simulink model "LAB4_interface_demo"  (R2023b)
settings: Solver=FixedStepAuto  StartTime=0.0  StopTime=inf  FixedStep=0.01  RelTol=1e-3
undefined symbols (not defined in the file or in its folder): LF
libraries: instrumentseriallib x4, simulink x3, hdlsllib x1
settings Model: Creator=tanawatp  LastModifiedBy=Kitti

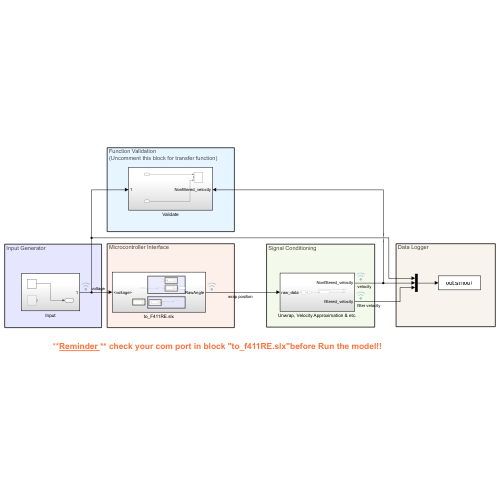
[thumbnail: Simulink's stored preview of the top-level diagram]
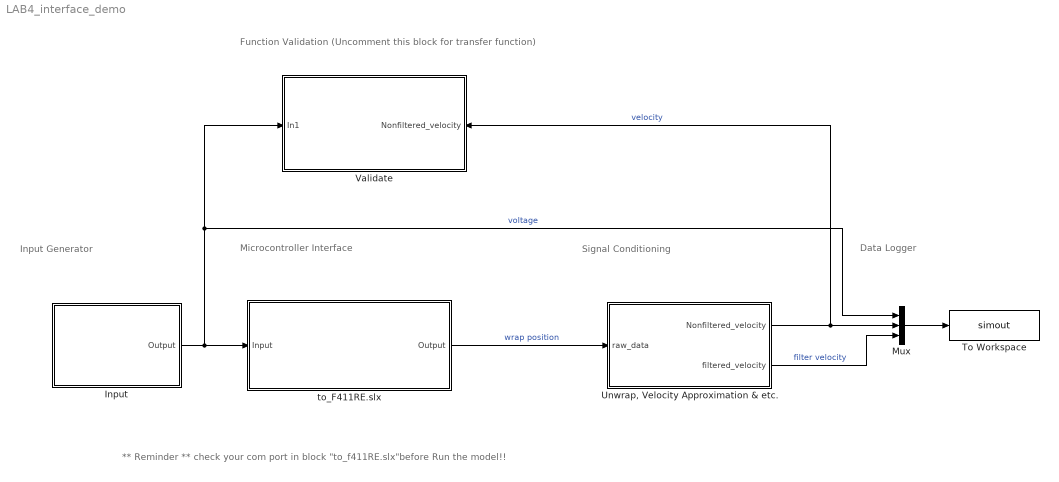
== system LAB4_interface_demo ==
  note: ** Reminder ** check your com port in block "to_f411RE.slx"before Run the model!!
  note: Signal Conditioning
  note: Function Validation
      | (Uncomment this block for transfer function)
  note: Input Generator
  note: Data Logger
  note: Microcontroller Interface
  Input : Subsystem
  Mux : Mux  Inputs=3
  To Workspace : ToWorkspace  VariableName=simout  SaveFormat=Timeseries  SampleTime=-1
  "Unwrap, Velocity Approximation & etc." : Subsystem
  Validate : Subsystem
      settings: PortSchema="{\"entries\":[{\"content\":{\"sides\":[{\"content\":{\"connectorIds\":[\"In1\"]},\"type\":\"ConnectorPlacement.EquallySpacedRectSide\",\"uuid\":\"2e198c62-3f63-40d2-bae8-9fd8fef67e0c\"},{\"content\":{\"connectorIds\":[\"In2\"],\"side\":\"RIGHT\"},\"type\":\"ConnectorPlacement.EquallySpacedRectSide\",\"uuid\":\"8587534e-14f7-4890-8a03-94178e65376b\"},{\"content\":{\"connectorIds\":[],\"side\":\"TOP\"},\"type\":\"ConnectorPlacement.EquallySpacedRectSide\",\"uuid\":\"1b7cad7c-cb5d-42c2-b7c5-a9278b867159\"}]},\"type\":\"ConnectorPlacement.EquallySpacedConnector\",\"uuid\":\"07c3edf9-7db3-4a0b-af16-87d57ef9c94a\"}],\"packageUris\":[\"http://schema.mathworks.com/mf0/Connector/R2020b\"],\"version\":\"1.0\"}"
  to_F411RE.slx : Subsystem
  wires:
  Mux/1 -> To Workspace/1
  to_F411RE.slx/1(Output) -> "Unwrap, Velocity Approximation & etc."/1(raw_data)  "wrap position"
  Input/1(Output) -> to_F411RE.slx/1(Input), Validate/1(In1), Mux/1  "voltage"
  "Unwrap, Velocity Approximation & etc."/1(Nonfiltered_velocity) -> Mux/2, Validate/2(Nonfiltered_velocity)  "velocity"
  "Unwrap, Velocity Approximation & etc."/2(filtered_velocity) -> Mux/3  "filter velocity"

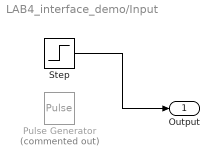
== system LAB4_interface_demo/Input ==
  Pulse Generator : DiscretePulseGenerator  Commented=on  PulseType=Time based  Amplitude=8  Period=5  PulseWidth=50  PhaseDelay=3
  Step : Step  After=6  SampleTime=0
  Output : Outport
  wires:
  Step/1 -> Output/1

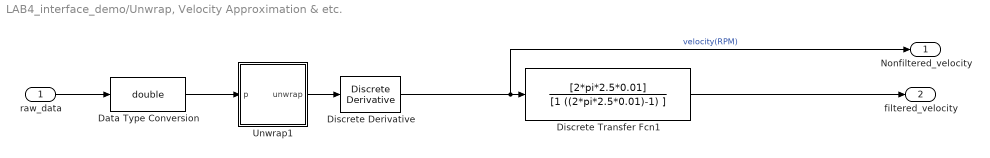
== system LAB4_interface_demo/Unwrap, Velocity Approximation & etc. ==
  raw_data : Inport
  Data Type Conversion : DataTypeConversion  OutDataTypeStr=double  SaturateOnIntegerOverflow=off  RndMeth=Floor
  Discrete Transfer Fcn1 : DiscreteTransferFcn  Numerator=[2*pi*2.5*0.01]  Denominator=[1 ((2*pi*2.5*0.01)-1) ]
  Discrete Derivative : simulink/Discrete/Discrete Derivative  gainval=60 / 4095  ICPrevScaledInput=0.0  OutMin=[]  OutMax=[]  OutDataType=fixdt(1, 16)  OutScaling=2^-10  DoSatur=off
  Unwrap1 : Subsystem
  Nonfiltered_velocity : Outport
  filtered_velocity : Outport  Port=2
  wires:
  Unwrap1/1(unwrap) -> Discrete Derivative/1
  raw_data/1 -> Data Type Conversion/1
  Discrete Transfer Fcn1/1 -> filtered_velocity/1
  Discrete Derivative/1 -> Nonfiltered_velocity/1, Discrete Transfer Fcn1/1  "velocity(RPM)"
  Data Type Conversion/1 -> Unwrap1/1(p)

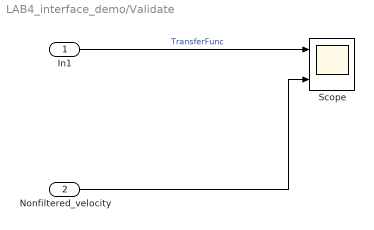
== system LAB4_interface_demo/Validate ==
  In1 : Inport
  Nonfiltered_velocity : Inport  Port=2
  Scope : Scope  NumInputPorts=3
  wires:
  Nonfiltered_velocity/1 -> Scope/3
  In1/1 -> Scope/1  "TransferFunc"

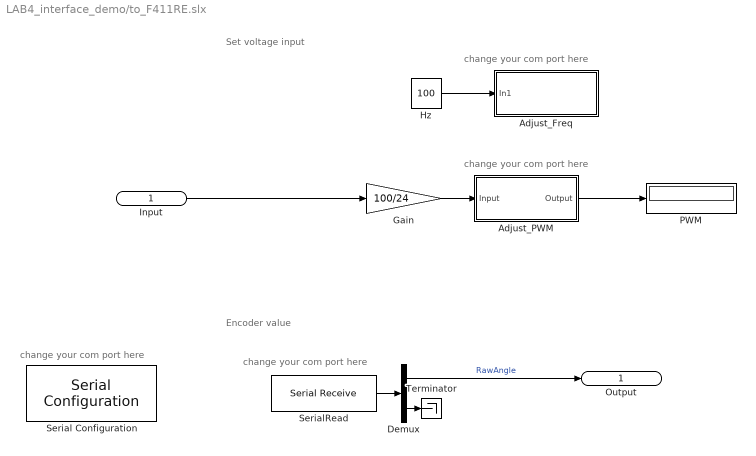
== system LAB4_interface_demo/to_F411RE.slx ==
  note: change your com port here
  note: Encoder value
  note: Set voltage input
  note: change your com port here
  note: change your com port here
  note: change your com port here
  Input : Inport
  Adjust_Freq : Subsystem
  Adjust_PWM : Subsystem
  Demux : Demux  Outputs=2
  Gain : Gain  Gain=100/24  OutDataTypeStr=int8
  Hz : Constant  Value=100  OutDataTypeStr=double
  PWM : Display
  Serial Configuration : instrumentseriallib/Serial Configuration  Priority=-200000  PortSel=COM5  Port=COM5  ComPort=COM5  BaudRate=115200  DataBits=8  Parity=none  StopBits=1  ByteOrder=little-endian  FlowControl=none  Timeout=10  SimulateUsing=Interpreted execution  BlockInModel=on  aMode=1
  SerialRead : instrumentseriallib/Serial Receive  Priority=1  PortSel=COM5  Port=COM5  ComPort=COM5  DataType=uint16  SaveDataType=uint8  ToggleHeader=on  Header=[69]  ToggleTerminator=on  Terminator=LF ('\n')  CustomTerminator=[]  InputFormat=Column major  ToggleDataSize=on  DataSize=[2]  EnableBlockingMode=on  ActionDataUnavailable=Output last received value  ActionWhenDataUnavailable=Output last received value  CustomValue=0  SampleTime=-1  SimulateUsing=Interpreted execution  BlockInModel=on  aMode=1
  Terminator : Terminator
  Output : Outport
  wires:
  Demux/1 -> Output/1  "RawAngle"
  Gain/1 -> Adjust_PWM/1(Input)
  Input/1 -> Gain/1
  Hz/1 -> Adjust_Freq/1(In1)
  Adjust_PWM/1(Output) -> PWM/1
  SerialRead/1 -> Demux/1
  Demux/2 -> Terminator/1

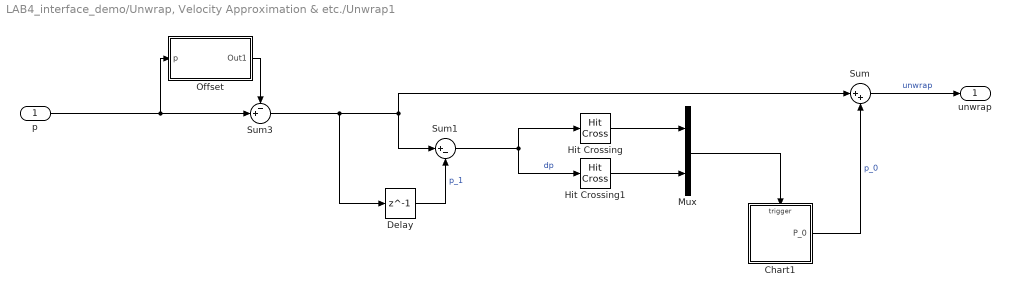
== system LAB4_interface_demo/Unwrap, Velocity Approximation & etc./Unwrap1 ==
  p : Inport
  Chart1 : Stateflow chart  TreatAsAtomicUnit=on
  Delay : Delay  DelayLength=1
  Hit Crossing : HitCross  HitCrossingOffset=0.7*65535  HitCrossingDirection=rising
  Hit Crossing1 : HitCross  HitCrossingOffset=-0.7*65535  HitCrossingDirection=falling
  Mux : Mux  Inputs=2
  Offset : Subsystem
  Sum : Sum  Inputs=|++
  Sum1 : Sum  Inputs=|+-
  Sum3 : Sum  Inputs=-+|
  unwrap : Outport
  wires:
  Hit Crossing/1 -> Mux/1
  Hit Crossing1/1 -> Mux/2
  Chart1/1(P_0) -> Sum/2  "p_0"
  Sum1/1 -> Hit Crossing1/1, Hit Crossing/1  "dp"
  Sum3/1 -> Delay/1, Sum/1, Sum1/1
  Mux/1 -> Chart1/Trigger
  Sum/1 -> unwrap/1  "unwrap"
  Delay/1 -> Sum1/2  "p_1"
  Offset/1(Out1) -> Sum3/1
  p/1 -> Sum3/2, Offset/1(p)

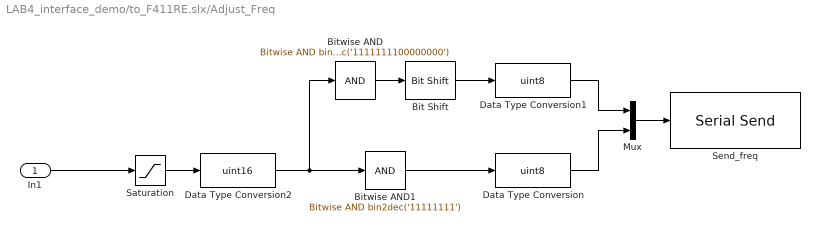
== system LAB4_interface_demo/to_F411RE.slx/Adjust_Freq ==
  In1 : Inport
  Bit Shift : hdlsllib/Logic and Bit Operations/Bit Shift  mode=Shift Right Logical  N=8
  Bitwise AND : simulink/Logic and Bit Operations/Bitwise Operator  logicop=AND  UseBitMask=on  BitMask=bin2dec('1111111100000000')  BitMaskRealWorld=Stored Integer
  Bitwise AND1 : simulink/Logic and Bit Operations/Bitwise Operator  logicop=AND  UseBitMask=on  BitMask=bin2dec('11111111')  BitMaskRealWorld=Stored Integer
  Data Type Conversion : DataTypeConversion  OutDataTypeStr=uint8  SaturateOnIntegerOverflow=off  RndMeth=Floor
  Data Type Conversion1 : DataTypeConversion  OutDataTypeStr=uint8  SaturateOnIntegerOverflow=off  RndMeth=Floor
  Data Type Conversion2 : DataTypeConversion  OutDataTypeStr=uint16  SaturateOnIntegerOverflow=off  RndMeth=Floor
  Mux : Mux  Inputs=2
  Saturation : Saturate  UpperLimit=20000  LowerLimit=5
  Send_freq : instrumentseriallib/Serial Send  Priority=1  PortSel=COM5  Port=COM5  ComPort=COM5  Header=[69]  Terminator=<none>  CustomTerminator=[123]  EnableBlockingMode=on  SimulateUsing=Interpreted execution  BlockInModel=on  aMode=1
  wires:
  Mux/1 -> Send_freq/1
  Saturation/1 -> Data Type Conversion2/1
  Data Type Conversion/1 -> Mux/2
  Bitwise AND/1 -> Bit Shift/1
  Bitwise AND1/1 -> Data Type Conversion/1
  Data Type Conversion2/1 -> Bitwise AND1/1, Bitwise AND/1
  Data Type Conversion1/1 -> Mux/1
  Bit Shift/1 -> Data Type Conversion1/1
  In1/1 -> Saturation/1

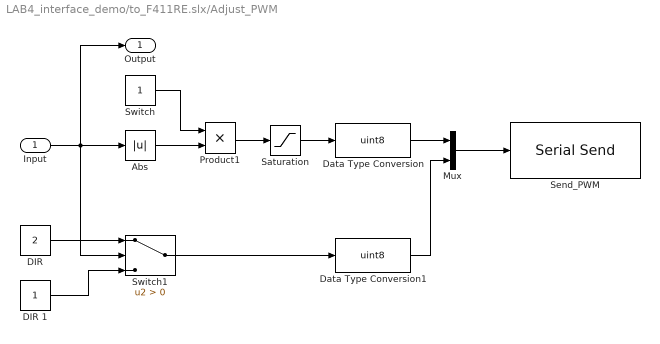
== system LAB4_interface_demo/to_F411RE.slx/Adjust_PWM ==
  Input : Inport
  Abs : Abs  SaturateOnIntegerOverflow=off
  "DIR " : Constant  Value=2
  DIR 1 : Constant
  Data Type Conversion : DataTypeConversion  OutDataTypeStr=uint8  SaturateOnIntegerOverflow=off  RndMeth=Floor
  Data Type Conversion1 : DataTypeConversion  OutDataTypeStr=uint8  SaturateOnIntegerOverflow=off  RndMeth=Floor
  Mux : Mux  Inputs=2
  Product1 : Product
  Saturation : Saturate  UpperLimit=200  LowerLimit=0
  Send_PWM : instrumentseriallib/Serial Send  Priority=1  PortSel=COM5  Port=COM5  ComPort=COM5  Header=[70]  Terminator=<none>  CustomTerminator=[123]  EnableBlockingMode=on  SimulateUsing=Interpreted execution  BlockInModel=on  aMode=1
  Switch : Constant
  Switch1 : Switch  Criteria=u2 > Threshold  SaturateOnIntegerOverflow=off  InputSameDT=off
  Output : Outport
  wires:
  Input/1 -> Switch1/2, Output/1, Abs/1
  Switch/1 -> Product1/1
  Product1/1 -> Saturation/1
  Data Type Conversion/1 -> Mux/1
  Saturation/1 -> Data Type Conversion/1
  Switch1/1 -> Data Type Conversion1/1
  Mux/1 -> Send_PWM/1
  Data Type Conversion1/1 -> Mux/2
  "DIR "/1 -> Switch1/1
  DIR 1/1 -> Switch1/3
  Abs/1 -> Product1/2

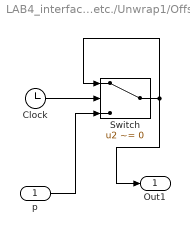
== system LAB4_interface_demo/Unwrap, Velocity Approximation & etc./Unwrap1/Offset ==
  p : Inport
  Clock : Clock
  Switch : Switch  Criteria=u2 ~= 0  SaturateOnIntegerOverflow=off  InputSameDT=off
  Out1 : Outport
  wires:
  Clock/1 -> Switch/2
  Switch/1 -> Out1/1, Switch/1
  p/1 -> Switch/3

== stateflow chart LAB4_interface_demo/Unwrap, Velocity Approximation & etc./Unwrap1/Chart1 ==
  settings: executeAtInitialization=1
  state initial
  (default) -> initial : {P_0 = 0;}
  initial -> initial [order 2] : e1{P_0 = P_0-65535;}
  initial -> initial [order 1] : e2{P_0 = P_0+65535;}
  data: P_0 output
  events: e1 input RISING_EDGE_EVENT; e2 input RISING_EDGE_EVENT
